simulink model "controlConDerivada"  (R2024b)
settings: Solver=VariableStepAuto  StartTime=0.0  StopTime=40.0  MaxStep=1e-2  RelTol=4
libraries: fuzblock x1
settings Model: Creator=juanp  LastModifiedBy=juanp

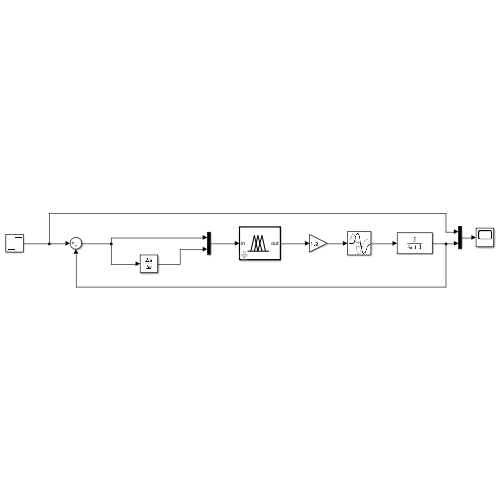
[thumbnail: Simulink's stored preview of the top-level diagram]
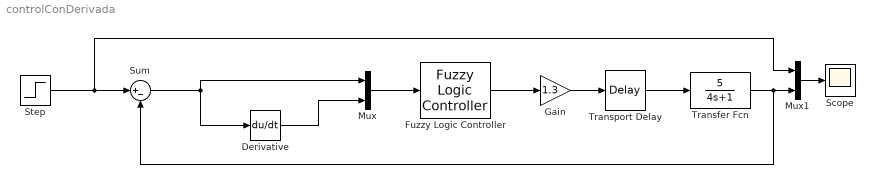
== system controlConDerivada ==
  Derivative : Derivative
  Fuzzy Logic Controller : fuzblock/Fuzzy Logic  Controller  FIS='controlPD.fis'  OutputSampleNumber=101  DataType=double  FuzzifiedInputs=off  RuleFiringStrengths=off  RuleOutputs=off  AggregatedOutputs=off  SimulateUsing=Interpreted execution  OutOfRangeInputValueMessage=warning  NoRuleFiredMessage=warning  EmptyOutputFuzzySetMessage=warning
  Gain : Gain  Gain=1.3
  Mux : Mux  Inputs=2
  Mux1 : Mux  Inputs=2
  Scope : Scope
  Step : Step  SampleTime=0
  Sum : Sum  Inputs=|+-
  Transfer Fcn : TransferFcn  Numerator=[5]  Denominator=[4 1]
  Transport Delay : TransportDelay  DelayTime=0.2
  wires:
  Step/1 -> Mux1/1, Sum/1
  Sum/1 -> Mux/1, Derivative/1
  Mux/1 -> Fuzzy Logic Controller/1
  Derivative/1 -> Mux/2
  Fuzzy Logic Controller/1 -> Gain/1
  Gain/1 -> Transport Delay/1
  Transport Delay/1 -> Transfer Fcn/1
  Transfer Fcn/1 -> Mux1/2, Sum/2
  Mux1/1 -> Scope/1
